simulink model "omnicopterTest"  (R2021a)
settings: Solver=VariableStepAuto  StartTime=0.0  StopTime=inf  RelTol=1e-3
values from neighbouring files (symbols this model uses):
  g = 10    [omnicopterStartUp.m]
  Ixx = 0.1    [omnicopterStartUp.m]
  l = 0.2    [omnicopterStartUp.m]
  m = 1    [omnicopterStartUp.m]
  phi = 0    [omnicopterStartUp.m]
  Ts = 0.1    [omnicopterStartUp.m]
  y = 0    [omnicopterStartUp.m]
  z = -5    [omnicopterStartUp.m]
undefined symbols (not defined in the file or in its folder): rl
libraries: simulink x5, vrlib x2, rllib x1
settings Model: Creator=da48y  LastModifiedBy=Psy

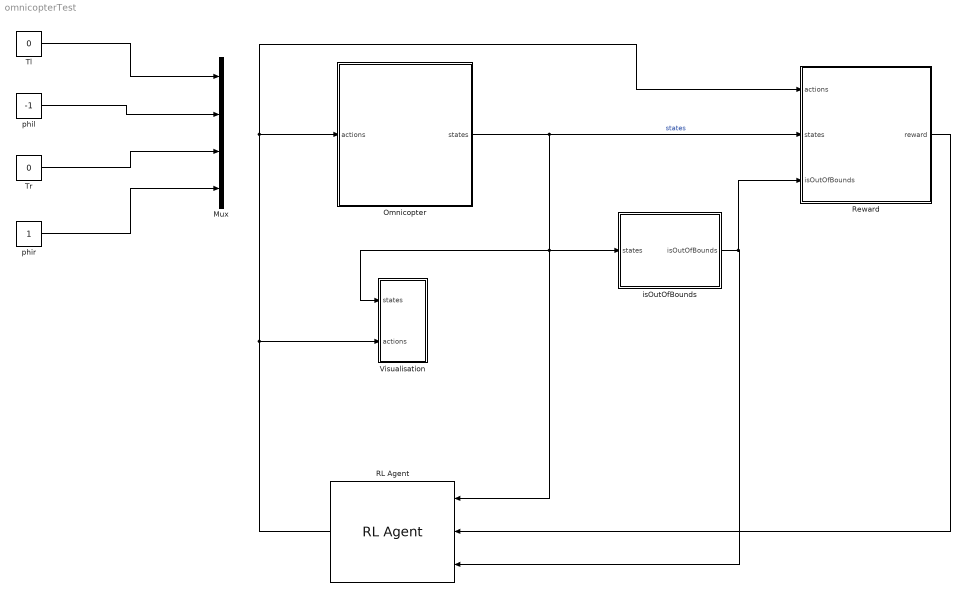
== system omnicopterTest ==
  Mux : Mux
  Omnicopter : Subsystem
  RL Agent : rllib/RL Agent  Agent=rl.util.PolicyInstance.get('omnicopterTest/RL Agent')  ExternalActionAsInput=off  ProvideCumRwd=off  TreatAsDirectFeedthrough=on
  Reward : Subsystem
  Tl : Constant  Value=0
  Tr : Constant  Value=0
  Visualisation : Subsystem
  isOutOfBounds : Subsystem
  phil : Constant  Value=-1
  phir : Constant
  wires:
  Omnicopter/1(states) -> RL Agent/1, isOutOfBounds/1(states), Visualisation/1(states), Reward/2(states)  "states"
  Tl/1 -> Mux/1
  phil/1 -> Mux/2
  Tr/1 -> Mux/3
  phir/1 -> Mux/4
  Reward/1(reward) -> RL Agent/2
  RL Agent/1 -> Visualisation/2(actions), Omnicopter/1(actions), Reward/1(actions)
  isOutOfBounds/1(isOutOfBounds) -> Reward/3(isOutOfBounds), RL Agent/3

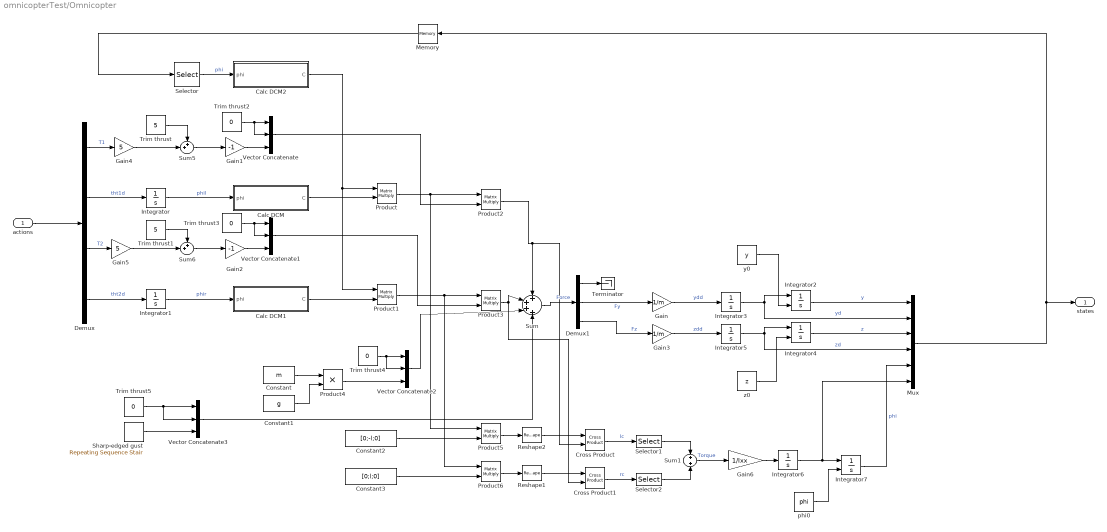
== system omnicopterTest/Omnicopter ==
  actions : Inport
  Calc DCM : MATLAB Function  TreatAsAtomicUnit=on
  Calc DCM1 : MATLAB Function  TreatAsAtomicUnit=on
  Calc DCM2 : MATLAB Function  TreatAsAtomicUnit=on
  Constant : Constant  Value=m
  Constant1 : Constant  Value=g
  Constant2 : Constant  Value=[0;-l;0]
  Constant3 : Constant  Value=[0;l;0]
  Cross Product : vrlib/Utilities/Cross Product
  Cross Product1 : vrlib/Utilities/Cross Product
  Demux : Demux
  Demux1 : Demux  Outputs=3
  Gain : Gain  Gain=1/m
  Gain1 : Gain  Gain=-1
  Gain2 : Gain  Gain=-1
  Gain3 : Gain  Gain=1/m
  Gain4 : Gain  Gain=5
  Gain5 : Gain  Gain=5
  Gain6 : Gain  Gain=1/Ixx
  Integrator{,1,3,5..6} (5 alike) : Integrator
  Integrator2 : Integrator  InitialConditionSource=external  InitialCondition=y
  Integrator4 : Integrator  InitialConditionSource=external  InitialCondition=z
  Integrator7 : Integrator  InitialConditionSource=external  InitialCondition=phi
  Memory : Memory
  Mux : Mux  Inputs=6
  Product{,1..3,5..6} (6 alike) : Product  Multiplication=Matrix(*)
  Product4 : Product
  Reshape1 : Reshape
  Reshape2 : Reshape
  Selector : Selector  InputPortWidth=6  IndexOptions=Index vector (dialog)  Indices=5  OutputSizes=1
  Selector1 : Selector  InputPortWidth=3  IndexOptions=Index vector (dialog)  Indices=1  OutputSizes=1
  Selector2 : Selector  InputPortWidth=3  IndexOptions=Index vector (dialog)  Indices=1  OutputSizes=1
  Sharp-edged gust : simulink/Sources/Repeating Sequence Stair  OutValues=[0 -2]  tsamp=2  OutMin=[]  OutMax=[]  OutDataTypeStr=double  OutputDataTypeScalingMode=double  OutDataType=fixdt(0,8)  ConRadixGroup=Best Precision: Vector-wise  OutScaling=2^-12
  Sum : Sum  Inputs=4
  Sum1 : Sum
  Sum5 : Sum  Inputs=++|
  Sum6 : Sum  Inputs=++|
  Terminator : Terminator
  Trim thrust : Constant  Value=5
  Trim thrust1 : Constant  Value=5
  Trim thrust{2..5} (4 alike) : Constant  Value=0
  Vector Concatenate{,1..3} (4 alike) : Concatenate  NumInputs=3
  phi0 : Constant  Value=phi
  y0 : Constant  Value=y
  z0 : Constant  Value=z
  states : Outport
  wires:
  Reshape1/1 -> Cross Product1/1
  Demux1/3 -> Gain3/1  "Fz"
  Integrator1/1 -> Calc DCM1/1(phi)  "phir"
  Product/1 -> Product5/1, Product2/1
  Vector Concatenate/1 -> Product2/2
  Gain3/1 -> Integrator5/1  "zdd"
  Integrator5/1 -> Mux/4, Integrator4/1  "zd"
  Memory/1 -> Selector/1
  Demux1/1 -> Terminator/1
  Product1/1 -> Product6/1, Product3/1
  Product3/1 -> Cross Product1/2, Sum/2
  Calc DCM2/1(C) -> Product1/1, Product/1
  Constant/1 -> Product4/1
  Vector Concatenate1/1 -> Product3/2
  Product4/1 -> Vector Concatenate2/3
  Integrator2/1 -> Mux/1  "y"
  Demux1/2 -> Gain/1  "Fy"
  Integrator7/1 -> Mux/5  "phi"
  Trim thrust1/1 -> Sum6/1
  Demux/2 -> Integrator/1  "tht1d"
  Gain5/1 -> Sum6/2
  actions/1 -> Demux/1
  Demux/4 -> Integrator1/1  "tht2d"
  Integrator/1 -> Calc DCM/1(phi)  "phil"
  Integrator4/1 -> Mux/3  "z"
  Constant1/1 -> Product4/2
  Demux/1 -> Gain4/1  "T1"
  Integrator3/1 -> Mux/2, Integrator2/1  "yd"
  Product5/1 -> Reshape2/1
  Integrator6/1 -> Mux/6, Integrator7/1
  Constant2/1 -> Product5/2
  Gain6/1 -> Integrator6/1
  Constant3/1 -> Product6/2
  Calc DCM1/1(C) -> Product1/2
  Sum5/1 -> Gain1/1
  Gain1/1 -> Vector Concatenate/3
  Sum/1 -> Demux1/1  "Force"
  Gain4/1 -> Sum5/2
  Demux/3 -> Gain5/1  "T2"
  Gain/1 -> Integrator3/1  "ydd"
  Sum6/1 -> Gain2/1
  Product2/1 -> Cross Product/2, Sum/1
  Reshape2/1 -> Cross Product/1
  Vector Concatenate2/1 -> Sum/3
  Gain2/1 -> Vector Concatenate1/3
  Product6/1 -> Reshape1/1
  Trim thrust2/1 -> Vector Concatenate/2, Vector Concatenate/1
  Trim thrust/1 -> Sum5/1
  Selector/1 -> Calc DCM2/1(phi)  "phi"
  Mux/1 -> Memory/1, states/1
  Trim thrust3/1 -> Vector Concatenate1/1, Vector Concatenate1/2
  Calc DCM/1(C) -> Product/2
  phi0/1 -> Integrator7/2
  z0/1 -> Integrator4/2
  y0/1 -> Integrator2/2
  Cross Product/1 -> Selector1/1  "lc"
  Cross Product1/1 -> Selector2/1  "rc"
  Sum1/1 -> Gain6/1  "Torque"
  Selector2/1 -> Sum1/2
  Selector1/1 -> Sum1/1
  Trim thrust4/1 -> Vector Concatenate2/2, Vector Concatenate2/1
  Vector Concatenate3/1 -> Sum/4
  Trim thrust5/1 -> Vector Concatenate3/2, Vector Concatenate3/1
  Sharp-edged gust/1 -> Vector Concatenate3/3

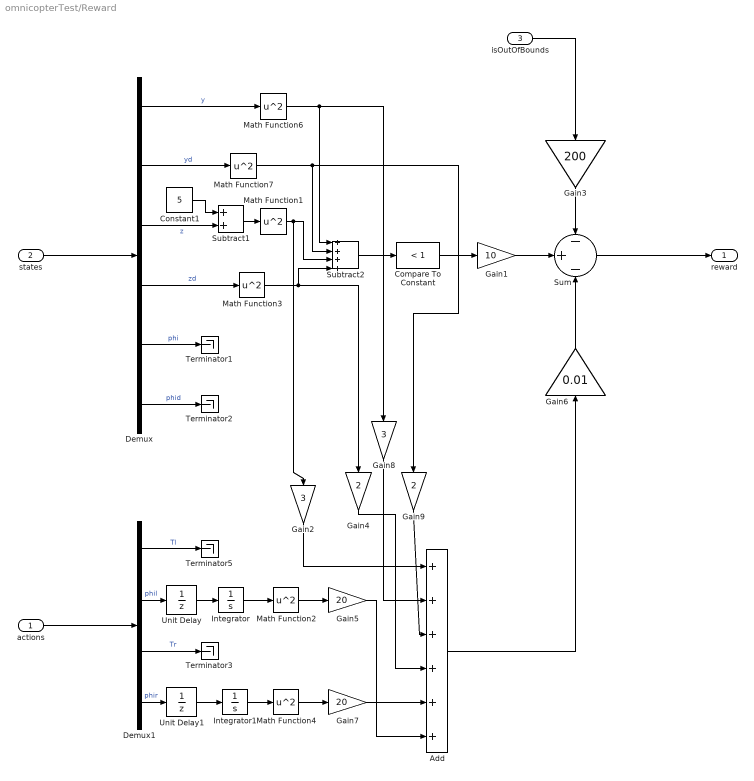
== system omnicopterTest/Reward ==
  actions : Inport
  states : Inport  Port=2
  isOutOfBounds : Inport  Port=3
  Add : Sum  Inputs=++++++
  Compare To Constant : simulink/Logic and Bit Operations/Compare To Constant  relop=<  const=1  OutDataTypeStr=boolean
  Constant1 : Constant  Value=5
  Demux : Demux  Outputs=6
  Demux1 : Demux
  Gain1 : Gain  Gain=10
  Gain2 : Gain  Gain=3
  Gain3 : Gain  Gain=200
  Gain4 : Gain  Gain=2
  Gain5 : Gain  Gain=20
  Gain6 : Gain  Gain=0.01
  Gain7 : Gain  Gain=20
  Gain8 : Gain  Gain=3
  Gain9 : Gain  Gain=2
  Integrator : Integrator
  Integrator1 : Integrator
  Math Function{1..4,6..7} (6 alike) : Math  Operator=square  SaturateOnIntegerOverflow=on
  Subtract1 : Sum
  Subtract2 : Sum  Inputs=++++
  Sum : Sum  Inputs=-+-
  Terminator{1..3,5} (4 alike) : Terminator
  Unit Delay : UnitDelay  SampleTime=Ts  HasFrameUpgradeWarning=on
  Unit Delay1 : UnitDelay  SampleTime=Ts  HasFrameUpgradeWarning=on
  reward : Outport
  wires:
  states/1 -> Demux/1
  Demux/6 -> Terminator2/1  "phid"
  Demux/1 -> Math Function6/1  "y"
  Demux/2 -> Math Function7/1  "yd"
  actions/1 -> Demux1/1
  Compare To Constant/1 -> Gain1/1
  Gain3/1 -> Sum/1
  isOutOfBounds/1 -> Gain3/1
  Gain1/1 -> Sum/2
  Add/1 -> Gain6/1
  Sum/1 -> reward/1
  Demux1/2 -> Unit Delay/1  "phil"
  Unit Delay/1 -> Integrator/1
  Demux1/4 -> Unit Delay1/1  "phir"
  Unit Delay1/1 -> Integrator1/1
  Math Function2/1 -> Gain5/1
  Math Function4/1 -> Gain7/1
  Math Function1/1 -> Subtract2/3, Gain2/1
  Constant1/1 -> Subtract1/1
  Demux/3 -> Subtract1/2  "z"
  Subtract1/1 -> Math Function1/1
  Subtract2/1 -> Compare To Constant/1
  Gain6/1 -> Sum/3
  Gain5/1 -> Add/6
  Gain7/1 -> Add/5
  Math Function6/1 -> Gain8/1, Subtract2/1
  Gain8/1 -> Add/2
  Gain9/1 -> Add/3
  Demux/4 -> Math Function3/1  "zd"
  Demux1/3 -> Terminator3/1  "Tr"
  Demux1/1 -> Terminator5/1  "Tl"
  Integrator/1 -> Math Function2/1
  Integrator1/1 -> Math Function4/1
  Gain2/1 -> Add/1
  Math Function3/1 -> Gain4/1, Subtract2/4
  Math Function7/1 -> Gain9/1, Subtract2/2
  Demux/5 -> Terminator1/1  "phi"
  Gain4/1 -> Add/4

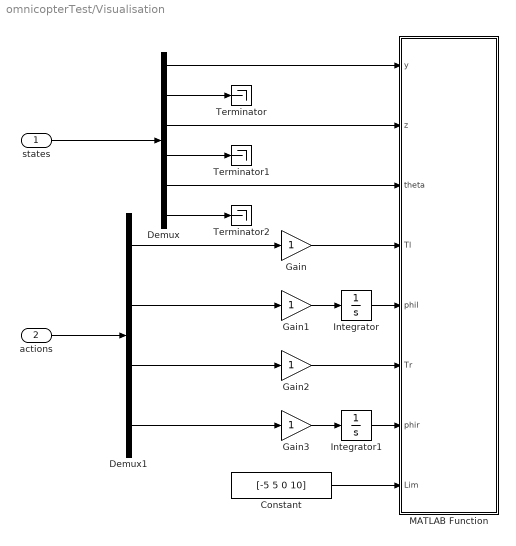
== system omnicopterTest/Visualisation ==
  states : Inport
  actions : Inport  Port=2
  Constant : Constant  Value=[-5 5 0 10]
  Demux : Demux  Outputs=6
  Demux1 : Demux
  Gain{,1..3} (4 alike) : Gain
  Integrator : Integrator
  Integrator1 : Integrator
  MATLAB Function : MATLAB Function  TreatAsAtomicUnit=on
  Terminator : Terminator
  Terminator1 : Terminator
  Terminator2 : Terminator
  wires:
  Integrator1/1 -> MATLAB Function/7(phir)
  Integrator/1 -> MATLAB Function/5(phil)
  Gain3/1 -> Integrator1/1
  Gain2/1 -> MATLAB Function/6(Tr)
  Gain1/1 -> Integrator/1
  Gain/1 -> MATLAB Function/4(Tl)
  Constant/1 -> MATLAB Function/8(Lim)
  Demux1/4 -> Gain3/1
  Demux1/3 -> Gain2/1
  Demux1/2 -> Gain1/1
  Demux1/1 -> Gain/1
  Demux/5 -> MATLAB Function/3(theta)
  Demux/3 -> MATLAB Function/2(z)
  Demux/1 -> MATLAB Function/1(y)
  Demux/6 -> Terminator2/1
  Demux/4 -> Terminator1/1
  Demux/2 -> Terminator/1
  actions/1 -> Demux1/1
  states/1 -> Demux/1

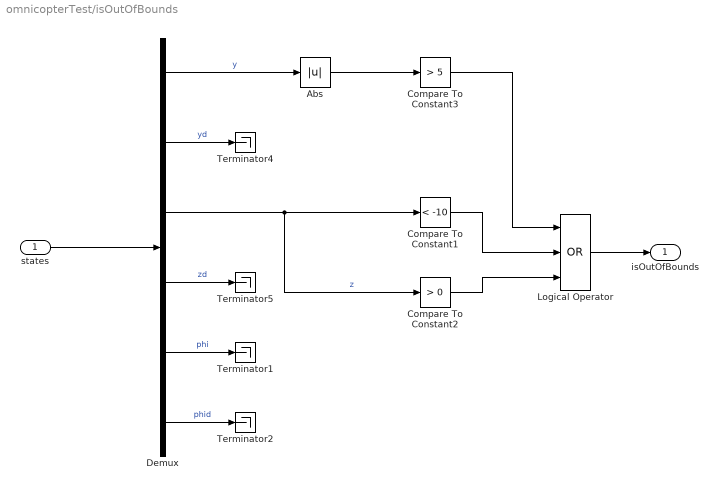
== system omnicopterTest/isOutOfBounds ==
  states : Inport
  Abs : Abs
  Compare To Constant1 : simulink/Logic and Bit Operations/Compare To Constant  relop=<  const=-10  OutDataTypeStr=boolean
  Compare To Constant2 : simulink/Logic and Bit Operations/Compare To Constant  relop=>  const=0  OutDataTypeStr=boolean
  Compare To Constant3 : simulink/Logic and Bit Operations/Compare To Constant  relop=>  const=5  OutDataTypeStr=boolean
  Demux : Demux  Outputs=6
  Logical Operator : Logic  Operator=OR  Inputs=3  AllPortsSameDT=off  OutDataTypeStr=boolean
  Terminator{1..2,4..5} (4 alike) : Terminator
  isOutOfBounds : Outport  VectorParamsAs1DForOutWhenUnconnected=off
  wires:
  Demux/1 -> Abs/1  "y"
  states/1 -> Demux/1
  Demux/5 -> Terminator1/1  "phi"
  Demux/2 -> Terminator4/1  "yd"
  Demux/6 -> Terminator2/1  "phid"
  Demux/4 -> Terminator5/1  "zd"
  Compare To Constant2/1 -> Logical Operator/3
  Compare To Constant1/1 -> Logical Operator/2
  Logical Operator/1 -> isOutOfBounds/1
  Demux/3 -> Compare To Constant1/1, Compare To Constant2/1  "z"
  Abs/1 -> Compare To Constant3/1
  Compare To Constant3/1 -> Logical Operator/1

== matlab function omnicopterTest/Visualisation/MATLAB Function ==
  data: y input; z input; theta input; Tl input; phil input; Tr input; phir input; Lim input
function fcn(y,z,theta,Tl,phil,Tr,phir,Lim)
%#codegen
coder.extrinsic('plotOmnicopter');
plotOmnicopter(y,z,theta,Tl,phil,Tr,phir,Lim);

== matlab function omnicopterTest/Omnicopter/Calc DCM ==
  data: phi input; C output
function C = fcn(phi)

C = [1 0 0;...
     0 cos(phi) -sin(phi);...
     0 sin(phi) cos(phi)];

== matlab function omnicopterTest/Omnicopter/Calc DCM1 ==
  data: phi input; C output
function C = fcn(phi)

C = [1 0 0;...
     0 cos(phi) -sin(phi);...
     0 sin(phi) cos(phi)];

== matlab function omnicopterTest/Omnicopter/Calc DCM2 ==
  data: phi input; C output
function C = fcn(phi)

C = [1 0 0;...
     0 cos(phi) -sin(phi);...
     0 sin(phi) cos(phi)];
